simulink model "example2"  (R2021b)
settings: Solver=FixedStepDiscrete  StartTime=0.0  StopTime=Tges  RelTol=1e-3
values from neighbouring files (symbols this model uses):
  Ts = simout.SimulationMetadata.ModelInfo.SolverInfo.FixedStepSize    [plot_phi.m]
libraries: simulink x1
settings Model: Creator=siegl  LastModifiedBy=siegl

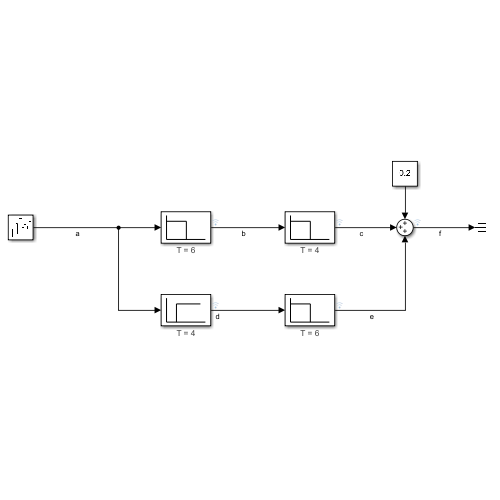
[thumbnail: Simulink's stored preview of the top-level diagram]
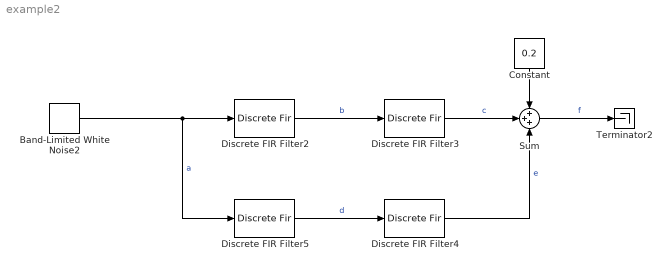
== system example2 ==
  Band-Limited White Noise2 : simulink/Sources/Band-Limited White Noise  Cov=2  Ts=Ts  seed=[23341]
  Constant : Constant  Value=0.2
  Discrete FIR Filter2 : DiscreteFir  Coefficients=ones(1,Tavg/SampleTime)*SampleTime/Tavg  SampleTime=SampleTime  mask{Tavg=6, SampleTime=Ts}
      mask prompts: Tavg "Average Time"; SampleTime "Simulink:blkprm_prompts:AllBlksSampleTime"
      settings: AttributesFormatString=T = %<Tavg>
      mask TypeOptions SampleTime: SampleTime
      mask DialogControl SampleTime Prompt: Sample time (-1 for inherited):
      mask Display:
      | plot([0.1, .9], [.1, .1])
      | plot([0.1, .1], [.1, .9])
      | plot([0.1, .5], [.7, .7])
      | plot([0.5, .5], [.7, .1])
  Discrete FIR Filter3 : DiscreteFir  Coefficients=ones(1,Tavg/SampleTime)*SampleTime/Tavg  SampleTime=SampleTime  mask{Tavg=4, SampleTime=Ts}
      mask prompts: Tavg "Average Time"; SampleTime "Simulink:blkprm_prompts:AllBlksSampleTime"
      settings: AttributesFormatString=T = %<Tavg>
      mask TypeOptions SampleTime: SampleTime
      mask DialogControl SampleTime Prompt: Sample time (-1 for inherited):
      mask Display:
      | plot([0.1, .9], [.1, .1])
      | plot([0.1, .1], [.1, .9])
      | plot([0.1, .5], [.7, .7])
      | plot([0.5, .5], [.7, .1])
  Discrete FIR Filter4 : DiscreteFir  Coefficients=ones(1,Tavg/SampleTime)*SampleTime/Tavg  SampleTime=SampleTime  mask{Tavg=6, SampleTime=Ts}
      mask prompts: Tavg "Average Time"; SampleTime "Simulink:blkprm_prompts:AllBlksSampleTime"
      settings: AttributesFormatString=T = %<Tavg>
      mask TypeOptions SampleTime: SampleTime
      mask DialogControl SampleTime Prompt: Sample time (-1 for inherited):
      mask Display:
      | plot([0.1, .9], [.1, .1])
      | plot([0.1, .1], [.1, .9])
      | plot([0.1, .5], [.7, .7])
      | plot([0.5, .5], [.7, .1])
  Discrete FIR Filter5 : DiscreteFir  Coefficients=[zeros(1,Td/SampleTime), 1]  SampleTime=SampleTime  mask{Td=4, SampleTime=Ts}
      mask prompts: Td "Delay Time"; SampleTime "Simulink:blkprm_prompts:AllBlksSampleTime"
      settings: AttributesFormatString=T = %<Td>
      mask TypeOptions SampleTime: SampleTime
      mask DialogControl SampleTime Prompt: Sample time (-1 for inherited):
      mask Display:
      | plot([0.1, .9], [.1, .1])
      | plot([0.1, .1], [.1, .9])
      | plot([0.3, .3], [.7, .1])
      | plot([0.3, .8], [.7, .7])
  Sum : Sum  Inputs=+++
  Terminator2 : Terminator
  wires:
  Discrete FIR Filter2/1 -> Discrete FIR Filter3/1  "b"
  Discrete FIR Filter5/1 -> Discrete FIR Filter4/1  "d"
  Discrete FIR Filter3/1 -> Sum/2  "c"
  Constant/1 -> Sum/1
  Sum/1 -> Terminator2/1  "f"
  Discrete FIR Filter4/1 -> Sum/3  "e"
  Band-Limited White Noise2/1 -> Discrete FIR Filter5/1, Discrete FIR Filter2/1  "a"
